simulink model "MBSE_Wind_Turbine"  (R2020a)
settings: Solver=VariableStepAuto  StartTime=0.0  StopTime=10.0  RelTol=1e-3
model workspace (MAT data in the model file):
  Aerodynamics_subsystem = Simulink.Bus
  Aerodynamics_subsystem.Alignment = -1
  Aerodynamics_subsystem.Elements_internal(1) = Simulink.BusElement
  Aerodynamics_subsystem.Elements_internal(1).Min_internal = 4
  Aerodynamics_subsystem.Elements_internal(1).Max_internal = 10
  Aerodynamics_subsystem.Elements_internal(1).DimensionsMode = 'Fixed'
  Aerodynamics_subsystem.Elements_internal(1).SamplingMode = 'Sample based'
  Aerodynamics_subsystem.Elements_internal(1).SampleTime = -1
  Aerodynamics_subsystem.Elements_internal(1).DocUnits = 'm/s'
  Aerodynamics_subsystem.Elements_internal(1).Name = 'Wind_speed'
  Aerodynamics_subsystem.Elements_internal(1).DataType_internal = 'double'
  Aerodynamics_subsystem.Elements_internal(1).Complexity = 'real'
  Aerodynamics_subsystem.Elements_internal(1).Dimensions = 1
  Aerodynamics_subsystem.Elements_internal(2) = Simulink.BusElement
  Aerodynamics_subsystem.Elements_internal(2).Min_internal = 0
  Aerodynamics_subsystem.Elements_internal(2).Max_internal = 360
  Aerodynamics_subsystem.Elements_internal(2).DimensionsMode = 'Fixed'
  Aerodynamics_subsystem.Elements_internal(2).SamplingMode = 'Sample based'
  Aerodynamics_subsystem.Elements_internal(2).SampleTime = -1
  Aerodynamics_subsystem.Elements_internal(2).DocUnits = 'deg/rad'
  Aerodynamics_subsystem.Elements_internal(2).Name = 'Wind_direction'
  Aerodynamics_subsystem.Elements_internal(2).DataType_internal = 'double'
  Aerodynamics_subsystem.Elements_internal(2).Complexity = 'real'
  Aerodynamics_subsystem.Elements_internal(2).Dimensions = 1
  Aerodynamics_subsystem.Elements_internal(3) = Simulink.BusElement
  Aerodynamics_subsystem.Elements_internal(3).Min_internal = 0
  Aerodynamics_subsystem.Elements_internal(3).Max_internal = 14
  Aerodynamics_subsystem.Elements_internal(3).DimensionsMode = 'Fixed'
  Aerodynamics_subsystem.Elements_internal(3).SamplingMode = 'Sample based'
  Aerodynamics_subsystem.Elements_internal(3).SampleTime = -1
  Aerodynamics_subsystem.Elements_internal(3).DocUnits = 'rpm'
  Aerodynamics_subsystem.Elements_internal(3).Name = 'Rotor_nominal_speed'
  Aerodynamics_subsystem.Elements_internal(3).DataType_internal = 'double'
  Aerodynamics_subsystem.Elements_internal(3).Complexity = 'real'
  Aerodynamics_subsystem.Elements_internal(3).Dimensions = 1
  Aerodynamics_subsystem.Elements_internal(4) = Simulink.BusElement
  Aerodynamics_subsystem.Elements_internal(4).DimensionsMode = 'Fixed'
  Aerodynamics_subsystem.Elements_internal(4).SamplingMode = 'Sample based'
  Aerodynamics_subsystem.Elements_internal(4).SampleTime = -1
  Aerodynamics_subsystem.Elements_internal(4).DocUnits = 'm'
  Aerodynamics_subsystem.Elements_internal(4).Name = 'Blade_length'
  Aerodynamics_subsystem.Elements_internal(4).DataType_internal = 'double'
  Aerodynamics_subsystem.Elements_internal(4).Complexity = 'real'
  Aerodynamics_subsystem.Elements_internal(4).Dimensions = 1
  Aerodynamics_subsystem.Elements_internal(5) = Simulink.BusElement
  Aerodynamics_subsystem.Elements_internal(5).DimensionsMode = 'Fixed'
  Aerodynamics_subsystem.Elements_internal(5).SamplingMode = 'Sample based'
  Aerodynamics_subsystem.Elements_internal(5).SampleTime = -1
  Aerodynamics_subsystem.Elements_internal(5).DocUnits = 'Nm'
  Aerodynamics_subsystem.Elements_internal(5).Name = 'Rotor_torque'
  Aerodynamics_subsystem.Elements_internal(5).DataType_internal = 'double'
  Aerodynamics_subsystem.Elements_internal(5).Complexity = 'real'
  Aerodynamics_subsystem.Elements_internal(5).Dimensions = 1
  Aerodynamics_subsystem.Elements_internal(6) = Simulink.BusElement
  Aerodynamics_subsystem.Elements_internal(6).DimensionsMode = 'Fixed'
  Aerodynamics_subsystem.Elements_internal(6).SamplingMode = 'Sample based'
  Aerodynamics_subsystem.Elements_internal(6).SampleTime = -1
  Aerodynamics_subsystem.Elements_internal(6).DocUnits = 'deg'
  Aerodynamics_subsystem.Elements_internal(6).Name = 'Desired_beta'
  Aerodynamics_subsystem.Elements_internal(6).DataType_internal = 'double'
  Aerodynamics_subsystem.Elements_internal(6).Complexity = 'real'
  Aerodynamics_subsystem.Elements_internal(6).Dimensions = 1
  Aerodynamics_subsystem.Elements_internal(7) = Simulink.BusElement
  Aerodynamics_subsystem.Elements_internal(7).DimensionsMode = 'Fixed'
  Aerodynamics_subsystem.Elements_internal(7).SamplingMode = 'Sample based'
  Aerodynamics_subsystem.Elements_internal(7).SampleTime = -1
  Aerodynamics_subsystem.Elements_internal(7).DocUnits = 'rpm'
  Aerodynamics_subsystem.Elements_internal(7).Name = 'Rotor_speed'
  Aerodynamics_subsystem.Elements_internal(7).DataType_internal = 'double'
  Aerodynamics_subsystem.Elements_internal(7).Complexity = 'real'
  Aerodynamics_subsystem.Elements_internal(7).Dimensions = 1
  Aerodynamics_subsystem.DataScope = 'Auto'
  Gear_train = Simulink.Bus
  Gear_train.Alignment = -1
  Gear_train.Elements_internal(1) = Simulink.BusElement
  Gear_train.Elements_internal(1).DimensionsMode = 'Fixed'
  Gear_train.Elements_internal(1).SamplingMode = 'Sample based'
  Gear_train.Elements_internal(1).SampleTime = -1
  Gear_train.Elements_internal(1).DocUnits = 'Nm'
  Gear_train.Elements_internal(1).Name = 'Generator_torque'
  Gear_train.Elements_internal(1).DataType_internal = 'double'
  Gear_train.Elements_internal(1).Complexity = 'real'
  Gear_train.Elements_internal(1).Dimensions = 1
  Gear_train.Elements_internal(2) = Simulink.BusElement
  Gear_train.Elements_internal(2).DimensionsMode = 'Fixed'
  Gear_train.Elements_internal(2).SamplingMode = 'Sample based'
  Gear_train.Elements_internal(2).SampleTime = -1
  Gear_train.Elements_internal(2).DocUnits = 'deg'
  Gear_train.Elements_internal(2).Name = 'Generator_speed'
  Gear_train.Elements_internal(2).DataType_internal = 'double'
  Gear_train.Elements_internal(2).Complexity = 'real'
  Gear_train.Elements_internal(2).Dimensions = 1
  Gear_train.DataScope = 'Auto'
  Pitch_subsystem = Simulink.Bus
  Pitch_subsystem.Alignment = -1
  Pitch_subsystem.Elements_internal = Simulink.BusElement
  Pitch_subsystem.Elements_internal.DimensionsMode = 'Fixed'
  Pitch_subsystem.Elements_internal.SamplingMode = 'Sample based'
  Pitch_subsystem.Elements_internal.SampleTime = -1
  Pitch_subsystem.Elements_internal.DocUnits = 'deg'
  Pitch_subsystem.Elements_internal.Name = 'A_beta'
  Pitch_subsystem.Elements_internal.DataType_internal = 'double'
  Pitch_subsystem.Elements_internal.Complexity = 'real'
  Pitch_subsystem.Elements_internal.Dimensions = 1
  Pitch_subsystem.DataScope = 'Auto'
  Yaw_subsystem = Simulink.Bus
  Yaw_subsystem.Alignment = -1
  Yaw_subsystem.Elements_internal = Simulink.BusElement
  Yaw_subsystem.Elements_internal.DimensionsMode = 'Fixed'
  Yaw_subsystem.Elements_internal.SamplingMode = 'Sample based'
  Yaw_subsystem.Elements_internal.SampleTime = -1
  Yaw_subsystem.Elements_internal.DocUnits = 'deg'
  Yaw_subsystem.Elements_internal.Name = 'A_theta'
  Yaw_subsystem.Elements_internal.DataType_internal = 'double'
  Yaw_subsystem.Elements_internal.Complexity = 'real'
  Yaw_subsystem.Elements_internal.Dimensions = 1
  Yaw_subsystem.DataScope = 'Auto'
settings Model: OrderedModelArguments=off  Creator=param  LastModifiedBy=param

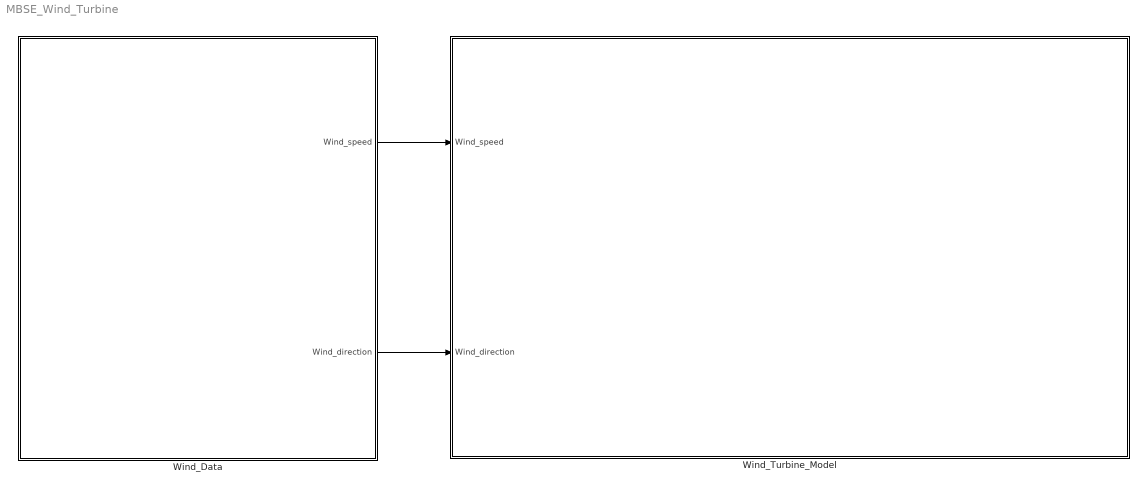
== system MBSE_Wind_Turbine ==
  Wind_Data : Subsystem
      settings: PortSchema="{\"entries\":[{\"content\":{\"headerSize\":26,\"margin\":15,\"minimumSpacing\":25,\"sides\":[{\"content\":{\"connectorIds\":[]},\"type\":\"ConnectorPlacement.EquallySpacedRectSide\",\"uuid\":\"0b654df8-291b-4ec3-b235-d9b2c2fe09d2\"},{\"content\":{\"connectorIds\":[\"Out1\",\"Out2\"],\"side\":\"RIGHT\"},\"type\":\"ConnectorPlacement.EquallySpacedRectSide\",\"uuid\":\"a4fe281e-c492-45bd-b5d6-a645186b9bb6\"},{\"content\":{\"connectorIds\":[],\"side\":\"TOP\"},\"type\":\"ConnectorPlacement.EquallySpacedRectSide\",\"uuid\":\"2d01dd3f-31b4-4e6a-a4ed-0a0bf71ed999\"}]},\"type\":\"ConnectorPlacement.EquallySpacedConnector\",\"uuid\":\"d70ff5d2-e302-4dc0-bd65-e713966bc3c0\"}],\"packageUris\":[\"http://schema.mathworks.com/mf0/Connector/19700101\"],\"version\":\"1.0\"}"
  Wind_Turbine_Model : Subsystem
      settings: PortSchema="{\"entries\":[{\"content\":{\"headerSize\":26,\"margin\":15,\"minimumSpacing\":25,\"sides\":[{\"content\":{\"connectorIds\":[\"In1\",\"In2\"]},\"type\":\"ConnectorPlacement.EquallySpacedRectSide\",\"uuid\":\"0b654df8-291b-4ec3-b235-d9b2c2fe09d2\"},{\"content\":{\"connectorIds\":[],\"side\":\"RIGHT\"},\"type\":\"ConnectorPlacement.EquallySpacedRectSide\",\"uuid\":\"a4fe281e-c492-45bd-b5d6-a645186b9bb6\"},{\"content\":{\"connectorIds\":[],\"side\":\"TOP\"},\"type\":\"ConnectorPlacement.EquallySpacedRectSide\",\"uuid\":\"2d01dd3f-31b4-4e6a-a4ed-0a0bf71ed999\"}]},\"type\":\"ConnectorPlacement.EquallySpacedConnector\",\"uuid\":\"d70ff5d2-e302-4dc0-bd65-e713966bc3c0\"}],\"packageUris\":[\"http://schema.mathworks.com/mf0/Connector/19700101\"],\"version\":\"1.0\"}"
  wires:
  Wind_Data/1(Wind_speed) -> Wind_Turbine_Model/1(Wind_speed)
  Wind_Data/2(Wind_direction) -> Wind_Turbine_Model/2(Wind_direction)

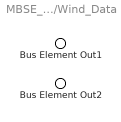
== system MBSE_Wind_Turbine/Wind_Data ==
  Bus Element Out1 : Outport  PortName=Wind_speed
  Bus Element Out2 : Outport  Port=2  PortName=Wind_direction

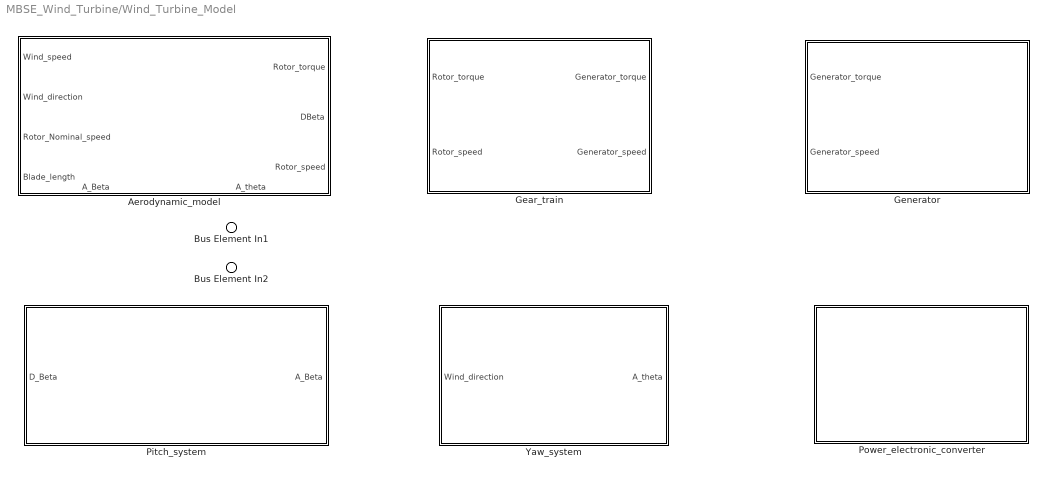
== system MBSE_Wind_Turbine/Wind_Turbine_Model ==
  Bus Element In1 : Inport  PortName=Wind_speed
  Bus Element In2 : Inport  Port=2  PortName=Wind_direction
  Aerodynamic_model : Subsystem
      settings: PortSchema="{\"entries\":[{\"content\":{\"headerSize\":26,\"margin\":15,\"minimumSpacing\":25,\"sides\":[{\"content\":{\"connectorIds\":[\"In5\",\"In6\",\"In3\",\"In4\"]},\"type\":\"ConnectorPlacement.EquallySpacedRectSide\",\"uuid\":\"0b654df8-291b-4ec3-b235-d9b2c2fe09d2\"},{\"content\":{\"connectorIds\":[\"Out1\",\"Out2\",\"Out3\"],\"side\":\"RIGHT\"},\"type\":\"ConnectorPlacement.EquallySpacedRectSide\",\"uuid\":\"a4fe281e-c492-45bd-b5d6-a645186b9bb6\"},{\"content\":{\"connectorIds\":[],\"side\":\"TOP\"},\"type\":\"ConnectorPlacement.EquallySpacedRectSide\",\"uuid\":\"2d01dd3f-31b4-4e6a-a4ed-0a0bf71ed999\"},{\"content\":{\"connectorIds\":[\"In1\",\"In2\"],\"side\":\"BOTTOM\"},\"type\":\"ConnectorPlacement.EquallySpacedRectSide\",\"uuid\":\"7a6130c0-1b48-47f4-9302-66f5dc87ee77\"}]},\"type\":\"ConnectorPlacement.EquallySpacedConnector\",\"uuid\":\"d70ff5d2-e302-4dc0-bd65-e713966bc3c0\"}],\"packageUris\":[\"http://schema.mathworks.com/mf0/Connector/19700101\"],\"version\":\"1.0\"}"
  Gear_train : Subsystem
      settings: PortSchema="{\"entries\":[{\"content\":{\"headerSize\":26,\"margin\":15,\"minimumSpacing\":25,\"sides\":[{\"content\":{\"connectorIds\":[\"In1\",\"In2\"]},\"type\":\"ConnectorPlacement.EquallySpacedRectSide\",\"uuid\":\"0b654df8-291b-4ec3-b235-d9b2c2fe09d2\"},{\"content\":{\"connectorIds\":[\"Out1\",\"Out2\"],\"side\":\"RIGHT\"},\"type\":\"ConnectorPlacement.EquallySpacedRectSide\",\"uuid\":\"a4fe281e-c492-45bd-b5d6-a645186b9bb6\"},{\"content\":{\"connectorIds\":[],\"side\":\"TOP\"},\"type\":\"ConnectorPlacement.EquallySpacedRectSide\",\"uuid\":\"2d01dd3f-31b4-4e6a-a4ed-0a0bf71ed999\"}]},\"type\":\"ConnectorPlacement.EquallySpacedConnector\",\"uuid\":\"d70ff5d2-e302-4dc0-bd65-e713966bc3c0\"}],\"packageUris\":[\"http://schema.mathworks.com/mf0/Connector/19700101\"],\"version\":\"1.0\"}"
  Generator : Subsystem
      settings: PortSchema="{\"entries\":[{\"content\":{\"headerSize\":26,\"margin\":15,\"minimumSpacing\":25,\"sides\":[{\"content\":{\"connectorIds\":[\"In1\",\"In2\"]},\"type\":\"ConnectorPlacement.EquallySpacedRectSide\",\"uuid\":\"0b654df8-291b-4ec3-b235-d9b2c2fe09d2\"},{\"content\":{\"connectorIds\":[],\"side\":\"RIGHT\"},\"type\":\"ConnectorPlacement.EquallySpacedRectSide\",\"uuid\":\"a4fe281e-c492-45bd-b5d6-a645186b9bb6\"},{\"content\":{\"connectorIds\":[],\"side\":\"TOP\"},\"type\":\"ConnectorPlacement.EquallySpacedRectSide\",\"uuid\":\"2d01dd3f-31b4-4e6a-a4ed-0a0bf71ed999\"}]},\"type\":\"ConnectorPlacement.EquallySpacedConnector\",\"uuid\":\"d70ff5d2-e302-4dc0-bd65-e713966bc3c0\"}],\"packageUris\":[\"http://schema.mathworks.com/mf0/Connector/19700101\"],\"version\":\"1.0\"}"
  Pitch_system : Subsystem
      settings: PortSchema="{\"entries\":[{\"content\":{\"headerSize\":26,\"margin\":15,\"minimumSpacing\":25,\"sides\":[{\"content\":{\"connectorIds\":[\"In1\"]},\"type\":\"ConnectorPlacement.EquallySpacedRectSide\",\"uuid\":\"0b654df8-291b-4ec3-b235-d9b2c2fe09d2\"},{\"content\":{\"connectorIds\":[\"Out1\"],\"side\":\"RIGHT\"},\"type\":\"ConnectorPlacement.EquallySpacedRectSide\",\"uuid\":\"a4fe281e-c492-45bd-b5d6-a645186b9bb6\"},{\"content\":{\"connectorIds\":[],\"side\":\"TOP\"},\"type\":\"ConnectorPlacement.EquallySpacedRectSide\",\"uuid\":\"2d01dd3f-31b4-4e6a-a4ed-0a0bf71ed999\"}]},\"type\":\"ConnectorPlacement.EquallySpacedConnector\",\"uuid\":\"d70ff5d2-e302-4dc0-bd65-e713966bc3c0\"}],\"packageUris\":[\"http://schema.mathworks.com/mf0/Connector/19700101\"],\"version\":\"1.0\"}"
  Power_electronic_converter : Subsystem
      settings: PortSchema="{\"entries\":[{\"content\":{\"headerSize\":26,\"margin\":15,\"minimumSpacing\":25,\"sides\":[{\"content\":{\"connectorIds\":[]},\"type\":\"ConnectorPlacement.EquallySpacedRectSide\",\"uuid\":\"0b654df8-291b-4ec3-b235-d9b2c2fe09d2\"},{\"content\":{\"connectorIds\":[],\"side\":\"RIGHT\"},\"type\":\"ConnectorPlacement.EquallySpacedRectSide\",\"uuid\":\"a4fe281e-c492-45bd-b5d6-a645186b9bb6\"},{\"content\":{\"connectorIds\":[],\"side\":\"TOP\"},\"type\":\"ConnectorPlacement.EquallySpacedRectSide\",\"uuid\":\"2d01dd3f-31b4-4e6a-a4ed-0a0bf71ed999\"}]},\"type\":\"ConnectorPlacement.EquallySpacedConnector\",\"uuid\":\"d70ff5d2-e302-4dc0-bd65-e713966bc3c0\"}],\"packageUris\":[\"http://schema.mathworks.com/mf0/Connector/19700101\"],\"version\":\"1.0\"}"
  Yaw_system : Subsystem
      settings: PortSchema="{\"entries\":[{\"content\":{\"headerSize\":26,\"margin\":15,\"minimumSpacing\":25,\"sides\":[{\"content\":{\"connectorIds\":[\"In1\"]},\"type\":\"ConnectorPlacement.EquallySpacedRectSide\",\"uuid\":\"0b654df8-291b-4ec3-b235-d9b2c2fe09d2\"},{\"content\":{\"connectorIds\":[\"Out1\"],\"side\":\"RIGHT\"},\"type\":\"ConnectorPlacement.EquallySpacedRectSide\",\"uuid\":\"a4fe281e-c492-45bd-b5d6-a645186b9bb6\"},{\"content\":{\"connectorIds\":[],\"side\":\"TOP\"},\"type\":\"ConnectorPlacement.EquallySpacedRectSide\",\"uuid\":\"2d01dd3f-31b4-4e6a-a4ed-0a0bf71ed999\"}]},\"type\":\"ConnectorPlacement.EquallySpacedConnector\",\"uuid\":\"d70ff5d2-e302-4dc0-bd65-e713966bc3c0\"}],\"packageUris\":[\"http://schema.mathworks.com/mf0/Connector/19700101\"],\"version\":\"1.0\"}"

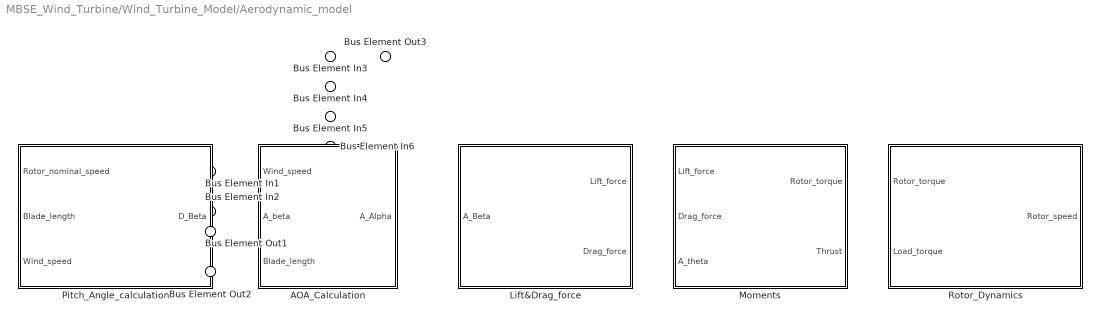
== system MBSE_Wind_Turbine/Wind_Turbine_Model/Aerodynamic_model ==
  Bus Element In3 : Inport  PortName=A_Beta
  Bus Element In4 : Inport  Port=2  PortName=A_theta
  Bus Element In5 : Inport  Port=3  PortName=Rotor_Nominal_speed
  Bus Element In6 : Inport  Port=4  PortName=Blade_length
  Bus Element In1 : Inport  Port=5  PortName=Wind_speed
  Bus Element In2 : Inport  Port=6  PortName=Wind_direction
  AOA_Calculation : Subsystem
      settings: PortSchema="{\"entries\":[{\"content\":{\"headerSize\":26,\"margin\":15,\"minimumSpacing\":25,\"sides\":[{\"content\":{\"connectorIds\":[\"In2\",\"Out1\",\"In3\"]},\"type\":\"ConnectorPlacement.EquallySpacedRectSide\",\"uuid\":\"ecf00de0-4a48-4b42-860b-7442add18d3c\"},{\"content\":{\"connectorIds\":[\"In1\"],\"side\":\"RIGHT\"},\"type\":\"ConnectorPlacement.EquallySpacedRectSide\",\"uuid\":\"09469086-fd43-4e9a-86e9-3abd2ebc91c2\"},{\"content\":{\"connectorIds\":[],\"side\":\"TOP\"},\"type\":\"ConnectorPlacement.EquallySpacedRectSide\",\"uuid\":\"5e523ea8-0f89-4af6-9d40-b6c57ace3a57\"}]},\"type\":\"ConnectorPlacement.EquallySpacedConnector\",\"uuid\":\"bd1a6e67-2730-4fcc-9b28-5e6f17ea94d8\"}],\"packageUris\":[\"http://schema.mathworks.com/mf0/Connector/19700101\"],\"version\":\"1.0\"}"
  Lift&Drag_force : Subsystem
      settings: PortSchema="{\"entries\":[{\"content\":{\"headerSize\":26,\"margin\":15,\"minimumSpacing\":25,\"sides\":[{\"content\":{\"connectorIds\":[\"In3\"]},\"type\":\"ConnectorPlacement.EquallySpacedRectSide\",\"uuid\":\"ecf00de0-4a48-4b42-860b-7442add18d3c\"},{\"content\":{\"connectorIds\":[\"In1\",\"In2\"],\"side\":\"RIGHT\"},\"type\":\"ConnectorPlacement.EquallySpacedRectSide\",\"uuid\":\"09469086-fd43-4e9a-86e9-3abd2ebc91c2\"},{\"content\":{\"connectorIds\":[],\"side\":\"TOP\"},\"type\":\"ConnectorPlacement.EquallySpacedRectSide\",\"uuid\":\"5e523ea8-0f89-4af6-9d40-b6c57ace3a57\"}]},\"type\":\"ConnectorPlacement.EquallySpacedConnector\",\"uuid\":\"bd1a6e67-2730-4fcc-9b28-5e6f17ea94d8\"}],\"packageUris\":[\"http://schema.mathworks.com/mf0/Connector/19700101\"],\"version\":\"1.0\"}"
  Moments : Subsystem
      settings: PortSchema="{\"entries\":[{\"content\":{\"headerSize\":26,\"margin\":15,\"minimumSpacing\":25,\"sides\":[{\"content\":{\"connectorIds\":[\"In4\",\"In5\",\"In3\"]},\"type\":\"ConnectorPlacement.EquallySpacedRectSide\",\"uuid\":\"ecf00de0-4a48-4b42-860b-7442add18d3c\"},{\"content\":{\"connectorIds\":[\"In1\",\"In2\"],\"side\":\"RIGHT\"},\"type\":\"ConnectorPlacement.EquallySpacedRectSide\",\"uuid\":\"09469086-fd43-4e9a-86e9-3abd2ebc91c2\"},{\"content\":{\"connectorIds\":[],\"side\":\"TOP\"},\"type\":\"ConnectorPlacement.EquallySpacedRectSide\",\"uuid\":\"5e523ea8-0f89-4af6-9d40-b6c57ace3a57\"}]},\"type\":\"ConnectorPlacement.EquallySpacedConnector\",\"uuid\":\"bd1a6e67-2730-4fcc-9b28-5e6f17ea94d8\"}],\"packageUris\":[\"http://schema.mathworks.com/mf0/Connector/19700101\"],\"version\":\"1.0\"}"
  Pitch_Angle_calculation : Subsystem
      settings: PortSchema="{\"entries\":[{\"content\":{\"headerSize\":26,\"margin\":15,\"minimumSpacing\":25,\"sides\":[{\"content\":{\"connectorIds\":[\"In2\",\"In4\",\"In3\"]},\"type\":\"ConnectorPlacement.EquallySpacedRectSide\",\"uuid\":\"ecf00de0-4a48-4b42-860b-7442add18d3c\"},{\"content\":{\"connectorIds\":[\"In1\"],\"side\":\"RIGHT\"},\"type\":\"ConnectorPlacement.EquallySpacedRectSide\",\"uuid\":\"09469086-fd43-4e9a-86e9-3abd2ebc91c2\"},{\"content\":{\"connectorIds\":[],\"side\":\"TOP\"},\"type\":\"ConnectorPlacement.EquallySpacedRectSide\",\"uuid\":\"5e523ea8-0f89-4af6-9d40-b6c57ace3a57\"}]},\"type\":\"ConnectorPlacement.EquallySpacedConnector\",\"uuid\":\"bd1a6e67-2730-4fcc-9b28-5e6f17ea94d8\"}],\"packageUris\":[\"http://schema.mathworks.com/mf0/Connector/19700101\"],\"version\":\"1.0\"}"
  Rotor_Dynamics : Subsystem
      settings: PortSchema="{\"entries\":[{\"content\":{\"headerSize\":26,\"margin\":15,\"minimumSpacing\":25,\"sides\":[{\"content\":{\"connectorIds\":[\"In2\",\"In3\"]},\"type\":\"ConnectorPlacement.EquallySpacedRectSide\",\"uuid\":\"ecf00de0-4a48-4b42-860b-7442add18d3c\"},{\"content\":{\"connectorIds\":[\"In1\"],\"side\":\"RIGHT\"},\"type\":\"ConnectorPlacement.EquallySpacedRectSide\",\"uuid\":\"09469086-fd43-4e9a-86e9-3abd2ebc91c2\"},{\"content\":{\"connectorIds\":[],\"side\":\"TOP\"},\"type\":\"ConnectorPlacement.EquallySpacedRectSide\",\"uuid\":\"5e523ea8-0f89-4af6-9d40-b6c57ace3a57\"}]},\"type\":\"ConnectorPlacement.EquallySpacedConnector\",\"uuid\":\"bd1a6e67-2730-4fcc-9b28-5e6f17ea94d8\"}],\"packageUris\":[\"http://schema.mathworks.com/mf0/Connector/19700101\"],\"version\":\"1.0\"}"
  Bus Element Out1 : Outport  PortName=Rotor_torque
  Bus Element Out3 : Outport  Port=2  PortName=DBeta
  Bus Element Out2 : Outport  Port=3  PortName=Rotor_speed

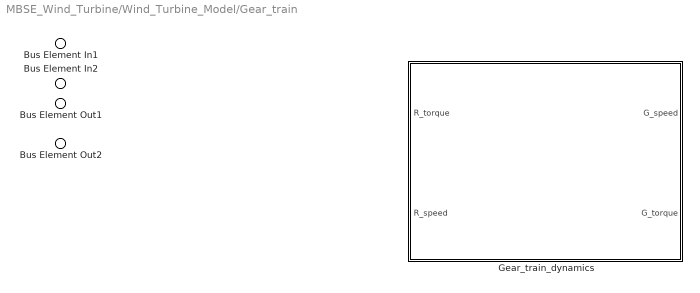
== system MBSE_Wind_Turbine/Wind_Turbine_Model/Gear_train ==
  Bus Element In1 : Inport  PortName=Rotor_torque
  Bus Element In2 : Inport  Port=2  PortName=Rotor_speed
  Gear_train_dynamics : Subsystem
      settings: PortSchema="{\"entries\":[{\"content\":{\"headerSize\":26,\"margin\":15,\"minimumSpacing\":25,\"sides\":[{\"content\":{\"connectorIds\":[\"In3\",\"In4\"]},\"type\":\"ConnectorPlacement.EquallySpacedRectSide\",\"uuid\":\"ecf00de0-4a48-4b42-860b-7442add18d3c\"},{\"content\":{\"connectorIds\":[\"In1\",\"In2\"],\"side\":\"RIGHT\"},\"type\":\"ConnectorPlacement.EquallySpacedRectSide\",\"uuid\":\"09469086-fd43-4e9a-86e9-3abd2ebc91c2\"},{\"content\":{\"connectorIds\":[],\"side\":\"TOP\"},\"type\":\"ConnectorPlacement.EquallySpacedRectSide\",\"uuid\":\"5e523ea8-0f89-4af6-9d40-b6c57ace3a57\"}]},\"type\":\"ConnectorPlacement.EquallySpacedConnector\",\"uuid\":\"bd1a6e67-2730-4fcc-9b28-5e6f17ea94d8\"}],\"packageUris\":[\"http://schema.mathworks.com/mf0/Connector/19700101\"],\"version\":\"1.0\"}"
  Bus Element Out1 : Outport  PortName=Generator_torque
  Bus Element Out2 : Outport  Port=2  PortName=Generator_speed

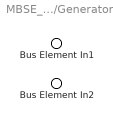
== system MBSE_Wind_Turbine/Wind_Turbine_Model/Generator ==
  Bus Element In1 : Inport  PortName=Generator_torque
  Bus Element In2 : Inport  Port=2  PortName=Generator_speed

== system MBSE_Wind_Turbine/Wind_Turbine_Model/Pitch_system ==
  Bus Element In1 : Inport  PortName=D_Beta
  Bus Element Out1 : Outport  PortName=A_Beta

== system MBSE_Wind_Turbine/Wind_Turbine_Model/Power_electronic_converter ==

== system MBSE_Wind_Turbine/Wind_Turbine_Model/Yaw_system ==
  Bus Element In1 : Inport  PortName=Wind_direction
  Bus Element Out1 : Outport  PortName=A_theta

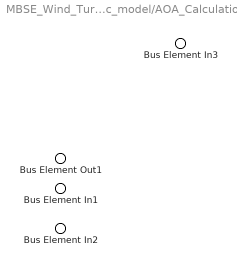
== system MBSE_Wind_Turbine/Wind_Turbine_Model/Aerodynamic_model/AOA_Calculation ==
  Bus Element In3 : Inport  PortName=A_Alpha
  Bus Element In1 : Inport  Port=2  PortName=Wind_speed
  Bus Element In2 : Inport  Port=3  PortName=Blade_length
  Bus Element Out1 : Outport  PortName=A_beta

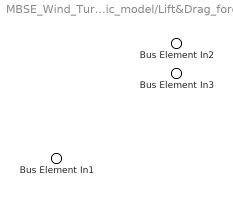
== system MBSE_Wind_Turbine/Wind_Turbine_Model/Aerodynamic_model/Lift&Drag_force ==
  Bus Element In2 : Inport  PortName=Lift_force
  Bus Element In3 : Inport  Port=2  PortName=Drag_force
  Bus Element In1 : Inport  Port=3  PortName=A_Beta

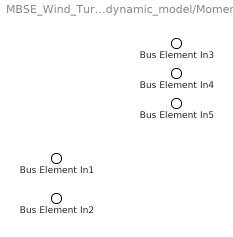
== system MBSE_Wind_Turbine/Wind_Turbine_Model/Aerodynamic_model/Moments ==
  Bus Element In3 : Inport  PortName=Rotor_torque
  Bus Element In4 : Inport  Port=2  PortName=Thrust
  Bus Element In5 : Inport  Port=3  PortName=A_theta
  Bus Element In1 : Inport  Port=4  PortName=Lift_force
  Bus Element In2 : Inport  Port=5  PortName=Drag_force

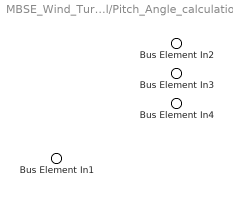
== system MBSE_Wind_Turbine/Wind_Turbine_Model/Aerodynamic_model/Pitch_Angle_calculation ==
  Bus Element In3 : Inport  PortName=D_Beta
  Bus Element In2 : Inport  Port=2  PortName=Rotor_nominal_speed
  Bus Element In4 : Inport  Port=3  PortName=Wind_speed
  Bus Element In1 : Inport  Port=4  PortName=Blade_length

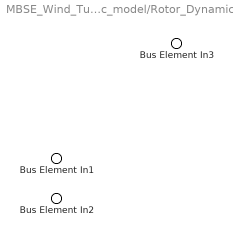
== system MBSE_Wind_Turbine/Wind_Turbine_Model/Aerodynamic_model/Rotor_Dynamics ==
  Bus Element In3 : Inport  PortName=Rotor_speed
  Bus Element In1 : Inport  Port=2  PortName=Rotor_torque
  Bus Element In2 : Inport  Port=3  PortName=Load_torque

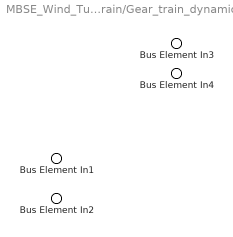
== system MBSE_Wind_Turbine/Wind_Turbine_Model/Gear_train/Gear_train_dynamics ==
  Bus Element In3 : Inport  PortName=G_speed
  Bus Element In4 : Inport  Port=2  PortName=G_torque
  Bus Element In1 : Inport  Port=3  PortName=R_torque
  Bus Element In2 : Inport  Port=4  PortName=R_speed
